simulink model "DTNS_SIM"  (R2022a)
settings: Solver=ode4  StartTime=0.0  StopTime=100  FixedStep=0.01  RelTol=1e-3
PreLoadFcn:
  | listing = dir;
  | if (contains([listing.name], 'MAP')) &&  (contains([listing.name], 'DTNS_SIM.slx'))
  |     addpath('./AGR', './TRN', './TCAF', './FTG', './DYN', './FLCC', './GPS', './RALT', './INS', './MAP');
  |     addpath('./MAP/MAP_DB');
  | else
  |     warning('[DTNS_SIM.slx]는 DTNS 프로젝트 최상단 경로에 위치해야 합니다.');
  | end
  | 
  | load('BUS_STRUCTURE_DYN.mat');
  | load('BUS_STRUCTURE_FLCC.mat');
  | load('BUS_STRUCTURE_RALT.mat');
  | load('BUS_STRUCTURE_INS.mat');
  | load('BUS_STRUCTURE_GPS.mat');
  | load('BusStructureTRN.mat');
  | load('BusStructureLOSR.mat');
  | load('BusStructureHR.mat');
  | load('BusStructureCR.mat');
  | FTG_initState;
InitFcn:
  | listing = dir;
  | if (contains([listing.name], 'MAP')) &&  (contains([listing.name], 'DTNS_SIM.slx'))
  |     addpath('./AGR', './TRN', './TCAF', './FTG', './DYN', './FLCC', './GPS', './RALT', './INS', './MAP');
  |     addpath('./MAP/MAP_DB');
  | else
  |     warning('[DTNS_SIM.slx]는 DTNS 프로젝트 최상단 경로에 위치해야 합니다.');
  | end
  | 
  | load('BUS_STRUCTURE_DYN.mat');
  | load('BUS_STRUCTURE_FLCC.mat');
  | load('BUS_STRUCTURE_RALT.mat');
  | load('BUS_STRUCTURE_INS.mat');
  | load('BUS_STRUCTURE_GPS.mat');
  | load('BusStructureTRN.mat');
  | load('BusStructureLOSR.mat');
  | load('BusStructureHR.mat');
  | load('BusStructureCR.mat');
  | FTG_initState;
undefined symbols (not defined in the file or in its folder): initState
libraries: aerolibconvert2 x16, simulink_extras x5
(part 2 of 2)

== matlab function DTNS_SIM/ControlFlightCmd ==
  data: inBus input Bus: BUS_FLCC_FLIGHT_CMD; outBus output Bus: BUS_FLCC_FLIGHT_CMD; state input Bus: BUS_DYN_STATE
function outBus = ControlFlightCmd(inBus, state)
%ControlFlightCmd
persistent time dt wayPoint
if isempty(time)
    time = 0.0;
end
if isempty(dt)
    dt = 0.01;
end
if isempty(wayPoint)
    wayPoint = 0;
end

ACTIVATED = true;

% -switchGCAS
SWICH_GCAS_NOT_SELECTED = uint8(0);
SWICH_GCAS_SELECTED     = uint8(1);
SWICH_GCAS_AUTO_GCAS    = uint8(2);

% -switchTF
SWICH_TF_NOT_SELECTED   = uint8(0);
SWICH_TF_SELECTED       = uint8(1);
SWICH_TF_AUTO_TF        = uint8(2);

% -switchRoll
SWITCH_ROLL_ATT_HOLD    = uint8(0);
SWITCH_ROLL_STRG_SEL    = uint8(1);
SWITCH_ROLL_HDG_SEL     = uint8(2);

% -switchPitch
SWITCH_PITCH_AP_OFF     = uint8(0);
SWITCH_PITCH_ATT_HOLD   = uint8(1);
SWITCH_PITCH_ALT_HOLD   = uint8(2);

% Copy
outBus = inBus;

if ACTIVATED
    
    % [Roll] Switch
%     outBus.switchRoll = SWITCH_ROLL_ATT_HOLD;
    outBus.switchRoll = SWITCH_ROLL_STRG_SEL;
%     outBus.switchRoll = SWITCH_ROLL_HDG_SEL;

    % [Pitch] Switch
%     outBus.switchPitch = SWITCH_PITCH_AP_OFF;
%     outBus.switchPitch = SWITCH_PITCH_ATT_HOLD;
    outBus.switchPitch = SWITCH_PITCH_ALT_HOLD;

    % [TF] Switch
%     outBus.switchTF = SWICH_TF_NOT_SELECTED;
%     outBus.switchTF = SWICH_TF_SELECTED;
    outBus.switchTF = SWICH_TF_AUTO_TF;

    % [GCAWS] Switch
%     outBus.switchGCAS = SWICH_GCAS_NOT_SELECTED;
    outBus.switchGCAS = SWICH_GCAS_SELECTED;
%     outBus.switchGCAS = SWICH_GCAS_AUTO_GCAS;

    % [WTPG] Sim: Roll
    %     outBus = SET_ATF(outBus, false, time, 0, inf);
    %     outBus = SET_ROLL_ATT(outBus, 30, time, 20, 20);
    %     outBus = SET_ROLL_ATT(outBus, -30, time, 40, 20);
    %     outBus = SET_ROLL_ATT(outBus, 0, time, 60, inf);

    % [DTF & GCAWS] Feasibility Sim
%     outBus.switchTF = SWICH_TF_SELECTED;
%     outBus.switchGCAS = SWICH_GCAS_AUTO_GCAS;
%     outBus.switchRoll = SWITCH_ROLL_ATT_HOLD;
    %     outBus.switchRoll = uint8(0);
    %     outBus.switchPitch = uint8(2);
    %     outBus.refSpeed = SET_VALUE(outBus.refSpeed, 100, time, 0, 40);
    %     outBus.refSpeed = SET_VALUE(outBus.refSpeed, 100, time, 40, 40);

        outBus.nextAlt = 900;
        outBus.refSpeed = 250;
        outBus.setHeading = 180;

    switch wayPoint
        case 0
            outBus.nextLat = 35.2;
            outBus.nextLon = 128;
        case 1
            outBus.nextLat = 34.8;
            outBus.nextLon = 128.4;
        case 2
            outBus.nextLat = 35.2;
            outBus.nextLon = 128.8;
        case 3
            outBus.nextLat = 37.0;
            outBus.nextLon = 129;
        otherwise
            outBus.nextLat = 37.0;
            outBus.nextLon = 129;
            outBus.nextAlt = 1000;
    end

    if ( abs(state.latitude - outBus.nextLat) < 0.001 ) && ( abs(state.longitude - outBus.nextLon) < 0.001 )
        wayPoint = wayPoint + 1;
    end

    %     outBus.nextAlt = 800.0;

end

% Update Time
time = time + dt;
end

function out = SET_ATF(in, isATF, curTime, triggerTime, duration)
% -switchTF
SWICH_TF_NOT_SELECTED   = uint8(0);
SWICH_TF_SELECTED       = uint8(1);
SWICH_TF_AUTO_TF        = uint8(2);

out = in;
if (triggerTime <= curTime) && (curTime <= triggerTime+duration)
    if isATF
        out.switchTF = SWICH_TF_AUTO_TF;
    else
        out.switchTF = SWICH_TF_SELECTED;
    end

else
end
end

function out = SET_ROLL_ATT(in, rollAngle, curTime, triggerTime, duration)
% -switchRoll
SWITCH_ROLL_ATT_HOLD    = uint8(0);
SWITCH_ROLL_STRG_SEL    = uint8(1);
SWITCH_ROLL_HDG_SEL     = uint8(2);

out = in;
if (triggerTime <= curTime) && (curTime <= triggerTime+duration)
    out.switchRoll = SWITCH_ROLL_ATT_HOLD;
    out.setRoll = rollAngle;
else
end
end

function out = SET_VALUE(in, value, curTime, triggerTime, duration)
out = in;
if (triggerTime <= curTime) && (curTime <= triggerTime+duration)
    out = value;
else
end
end

== matlab function DTNS_SIM/ControlCREvent ==
  data: outBus output Bus: CRInput; inBus input Bus: CRInput
function outBus  = ControlCREvent(inBus)
%ControlCREvent
persistent time dt
if isempty(time)
    time = 0.0;
end
if isempty(dt)
    dt = 0.04;
end

ACTIVATED = false;

% Copy
outBus   = inBus;

if ACTIVATED

%     outBus.CRSelected = SET_VALUE(inBus.CRSelected, false, time, 55, 1);

end


time = time + dt;
end


function out = SET_VALUE(in, value, curTime, triggerTime, duration)
out = in;
if (triggerTime <= curTime) && (curTime <= triggerTime+duration)
    out = value;
else
end
end

== matlab function DTNS_SIM/ControlGCAWSInput ==
  data: inBus input Bus: GCAWSInput; GCAWWSInput output Bus: GCAWSInput
function GCAWWSInput = ControlGCAWSInput(inBus)
%ControlGCAWSInput
persistent time dt
if isempty(time)
    time = 0.0;
end
if isempty(dt)
    dt = 0.01;
end
% -------------------------------------------------------------------------
% CONTROL flag
CONTROL_ACTIVATED = true;

% Copy
GCAWWSInput = inBus;

if CONTROL_ACTIVATED
    % Default
    GCAWWSInput.selected            = SET_VALUE(GCAWWSInput.selected,       true, time, 0, inf);
    GCAWWSInput.paramSelected       = SET_VALUE(GCAWWSInput.paramSelected,  true, time, 0, inf);
    GCAWWSInput.reactionTime        = SET_VALUE(GCAWWSInput.reactionTime,       uint16(3), time, 0, inf);
    GCAWWSInput.rollRate            = SET_VALUE(GCAWWSInput.rollRate,           uint16(3), time, 0, inf);
    GCAWWSInput.gOnsetRate          = SET_VALUE(GCAWWSInput.gOnsetRate,         uint16(3), time, 0, inf);
    GCAWWSInput.pullUpG             = SET_VALUE(GCAWWSInput.pullUpG,            uint16(3), time, 0, inf);
    GCAWWSInput.maxFlightPathAngle  = SET_VALUE(GCAWWSInput.maxFlightPathAngle, uint16(2), time, 0, inf);
    GCAWWSInput.gsAvailable         = SET_VALUE(GCAWWSInput.gsAvailable,        5.0, time, 0, inf);
    GCAWWSInput.gsAvaliableValid    = SET_VALUE(GCAWWSInput.gsAvaliableValid,   true, time, 0, inf);
    GCAWWSInput.swh                 = SET_VALUE(GCAWWSInput.swh,                single(500), time, 0, inf);

    % Control
%     outBus.msd = SET_VALUE(outBus.msd, 500, time, 100, 50);
%     outBus.msd = SET_VALUE(outBus.msd, 500, time, 200, 50);

end

% Update Time
time = time + dt;
end

function out = SET_VALUE(in, value, curTime, triggerTime, duration)
out = in;
if (triggerTime <= curTime) && (curTime <= triggerTime+duration)
    out = value;
else
end
end

== matlab function DTNS_SIM/ControlTFInput ==
  data: inBus input Bus: DTFInput; DTFInput output Bus: DTFInput; RALTDatapumpPrev input
function DTFInput = ControlTFInput(inBus, RALTDatapumpPrev)
%ControlTFInput
persistent time dt
if isempty(time)
    time = 0.0;
end
if isempty(dt)
    dt = 0.01;
end
% -------------------------------------------------------------------------
% CONTROL flag
CONTROL_ACTIVATED = true;

% Copy
DTFInput = inBus;

if CONTROL_ACTIVATED
    % Default
    DTFInput.selected   = SET_VALUE(DTFInput.selected, true, time, 0, inf);
    DTFInput.rideQuality= SET_VALUE(DTFInput.rideQuality, uint16(3), time, 0, inf);
    DTFInput.msd        = SET_VALUE(DTFInput.msd, 500, time, 0, inf);
    DTFInput.raltValid  = SET_VALUE(DTFInput.raltValid, RALTDatapumpPrev.RadarAltitudeValid, time, 0, inf);
    DTFInput.raltAlt    = SET_VALUE(DTFInput.raltAlt, RALTDatapumpPrev.RadarAltitude, time, 0, inf);

    % Control
%     outBus.msd = SET_VALUE(outBus.msd, 500, time, 100, 50);
%     outBus.msd = SET_VALUE(outBus.msd, 500, time, 200, 50);

end

% Update Time
time = time + dt;
end

function out = SET_VALUE(in, value, curTime, triggerTime, duration)
out = in;
if (triggerTime <= curTime) && (curTime <= triggerTime+duration)
    out = value;
else
end
end

== matlab function DTNS_SIM/TRNDataProcess/Subsystem3/Flag_WoW ==
  data: time input; WeightOnWheels output
function WeightOnWheels  = fcn(time)

% WeightOnWheels
% False[0]_flight / True[1]_ground

% if time <= 30
if time < 0
    WeightOnWheels = boolean(true);
else
    WeightOnWheels = boolean(false);
end

end

== matlab function DTNS_SIM/TRNDataProcess/Subsystem3/MATLAB Function ==
  data: count input; count output
function count = fcn(count)

count = count + 0.04;

== matlab function DTNS_SIM/TRNDataProcess/Subsystem3/Subsystem1/MATLAB Function1 ==
  data: WoW input; time input; lat_bias output; lon_bias output
function [lat_bias,lon_bias] = fcn(WoW, time)
%% parameters
lat2m = 111000;
lon2m = 91170;
bias1 = 0;   % 500m
bias2 = 0;   % 500m


%%
% if time > 60
if time >= 0
    if WoW == 0                % 0_flight / 1_ground
        lat_bias = bias1/lat2m;
        lon_bias = bias2/lon2m;
    else
        lat_bias = 0;
        lon_bias = 0;
    end
else
    lat_bias = 0;
    lon_bias = 0;
end

== matlab function DTNS_SIM/TRNDataProcess/Subsystem3/Subsystem1/MATLAB Function3 ==
  data: u input; a output; b output
function [a,b]  = fcn(u)

% WeightOnWheels
if(u==1)
    a = boolean(true);
    b = boolean(true);
else
    a = boolean(false);
    b = boolean(false);
end

end
